simulink model "fsk_matlab"  (R2022b)
settings: Solver=VariableStepAuto  StartTime=0.0  StopTime=5  RelTol=1e-3
libraries: commsynccomp2 x1
settings Model: Creator=saatt  LastModifiedBy=saatt

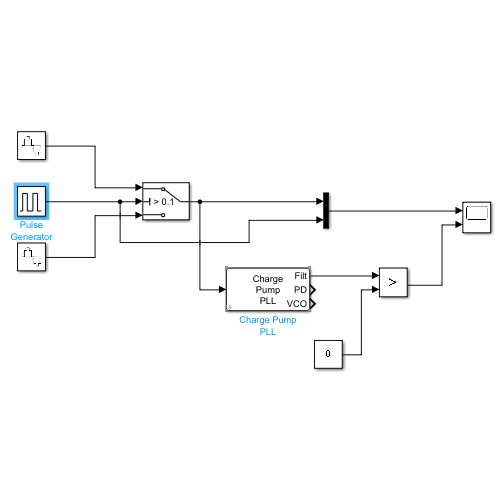
[thumbnail: Simulink's stored preview of the top-level diagram]
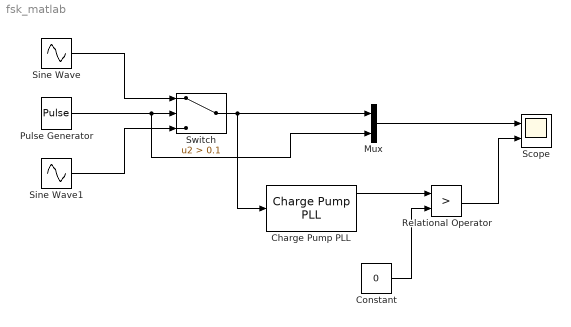
== system fsk_matlab ==
  Charge Pump PLL : commsynccomp2/Charge Pump PLL  Fn=[2*pi*1]  Fd="[1   2*pi*1]"  Kvco=4  Fc=8  Ph=0  Ac=1
  Constant : Constant  Value=0
  Mux : Mux  Inputs=2
  Pulse Generator : DiscretePulseGenerator  PulseType=Time based  Period=1  PulseWidth=50
  Relational Operator : RelationalOperator  Operator=>  OutDataTypeStr=boolean  RndMeth=Simplest  InputSameDT=off
  Scope : Scope  NumInputPorts=2
  Sine Wave : Sin  Frequency=2*pi*12  SampleTime=0.001
  Sine Wave1 : Sin  Frequency=2*pi*4  SampleTime=0.001
  Switch : Switch  Criteria=u2 > Threshold  Threshold=0.1  SaturateOnIntegerOverflow=off  InputSameDT=off
  wires:
  Pulse Generator/1 -> Mux/2, Switch/2
  Sine Wave/1 -> Switch/1
  Sine Wave1/1 -> Switch/3
  Mux/1 -> Scope/1
  Switch/1 -> Charge Pump PLL/1, Mux/1
  Charge Pump PLL/1 -> Relational Operator/1
  Constant/1 -> Relational Operator/2
  Relational Operator/1 -> Scope/2
